simulink model "peacockElettricaSimulink2025b"  (R2025b)
settings: Solver=FixedStepAuto  StopTime=30  FixedStep=0.001  MaxStep=0.001
InitFcn:
  | run('setupParams.m');
StopFcn:
  | plot(out.X, out.Y); axis equal; grid on;
model workspace: external: MATLAB File (data not in the file)
values from neighbouring files (symbols this model uses):
  air_temp = 300    [setupParams.m]    (also in setupParamsSingle.m)
  brake_bias_f = 0.60    (= 0.6)    [setupParams.m]    (also in setupParamsSingle.m)
  brake_bias_r = 1 - brake_bias_f    (= 0.4)    [setupParams.m]    (also in setupParamsSingle.m)
  camber_front = -1.5    [setupParams.m]    (also in setupParamsSingle.m)
  camber_rear = -1    [setupParams.m]    (also in setupParamsSingle.m)
  g = 9.81    [setupParams.m]    (also in setupParamsSingle.m)
  gnd_displ = 0.0    (= 0)    [setupParams.m]    (also in setupParamsSingle.m)
  Kus = 0.00    (= 0)    [setupParams.m]    (also in setupParamsSingle.m)
  l_f = 0.775    [setupParams.m]    (also in setupParamsSingle.m)
  l_r = 0.775    [setupParams.m]    (also in setupParamsSingle.m)
  launch_ramp_rate = 1000.0    (= 1000)    [setupParams.m]    (also in setupParamsSingle.m)
  launch_V_thresh = 5.0    (= 5)    [setupParams.m]    (also in setupParamsSingle.m)
  mass = 300    [setupParams.m]    (also in setupParamsSingle.m)
  mu = 1.5    [setupParams.m]    (also in setupParamsSingle.m)
  nominal_ramp_rate = 1000.0    (= 1000)    [setupParams.m]    (also in setupParamsSingle.m)
  pa_front_wheel = 82700    [setupParams.m]    (also in setupParamsSingle.m)
  pa_rear_wheel = 82700    [setupParams.m]    (also in setupParamsSingle.m)
  pedal_bp = (0:10:100)'    [setupParams.m]    (also in setupParamsSingle.m)
  pedal_map = (pedal_bp / 100) .^ pedal_alpha    [setupParams.m]    (also in setupParamsSingle.m = (pedal_bp / 100) .^ pedal_alpha.Value)
  R_wheel = 0.2032    [setupParams.m]    (also in setupParamsSingle.m)
  regen_I_cont_A = 14.0    (= 14)    [setupParams.m]    (also in setupParamsSingle.m)
  regen_I_peak_A = 21.0    (= 21)    [setupParams.m]    (also in setupParamsSingle.m)
  regen_I_peak_dur_s = 4.0    (= 4)    [setupParams.m]    (also in setupParamsSingle.m)
  regen_P_batt_max_W = 35000    [setupParams.m]    (also in setupParamsSingle.m)
  regen_pedal_thr = 10.0    (= 10)    [setupParams.m]    (also in setupParamsSingle.m)
  regen_speed_crit_rpm = 2000    [setupParams.m]    (also in setupParamsSingle.m = 500)
  regen_speed_min_rpm = 4000    [setupParams.m]    (also in setupParamsSingle.m = 3000)
  regen_T_max = 5    [setupParams.m]    (also in setupParamsSingle.m = Simulink.Parameter(T_rated.Value/2))
  rid_eff = 0.80    (= 0.8)    [setupParams.m]    (also in setupParamsSingle.m)
  rid_ratio = 15    [setupParams.m]    (also in setupParamsSingle.m)
  scale_factor_front = ones(27, 1)    [setupParams.m]    (also in setupParamsSingle.m)
  scale_factor_rear = ones(27, 1)    [setupParams.m]    (also in setupParamsSingle.m)
  slc_Ki = 0    [setupParams.m]    (also in setupParamsSingle.m = Simulink.Parameter(0))
  slc_Kp = 0    [setupParams.m]    (also in setupParamsSingle.m = Simulink.Parameter(0))
  slc_low_sat = -T_peak    (= -21)    [setupParams.m]    (also in setupParamsSingle.m)
  slc_up_sat = T_peak    (= 21)    [setupParams.m]    (also in setupParamsSingle.m)
  slip_bc_coeff = 10    [setupParams.m]    (also in setupParamsSingle.m = Simulink.Parameter(1.5))
  slip_filt_N = 80    [setupParams.m]    (also in setupParamsSingle.m = 15)
  slip_Kd = 0.8    [setupParams.m]    (also in setupParamsSingle.m = Simulink.Parameter(5.0))
  slip_Ki = 13.0    (= 13)    [setupParams.m]    (also in setupParamsSingle.m = Simulink.Parameter(110.0))
  slip_Kp = 50.0    (= 50)    [setupParams.m]    (also in setupParamsSingle.m = Simulink.Parameter(180.0))
  slip_low_sat = 0.0    (= 0)    [setupParams.m]    (also in setupParamsSingle.m)
  slip_ref = 0.15    [setupParams.m]    (also in setupParamsSingle.m = Simulink.Parameter(0.15))
  slip_up_sat = 18    [setupParams.m]    (also in setupParamsSingle.m = 21)
  slip_V_min = 3    [setupParams.m]    (also in setupParamsSingle.m = 1)
  steer_ratio = 4.2    [pure_pursuit.m]    (also in setupParams.m; setupParamsSingle.m)
  T_headroom_max = 3.0    (= 3)    [setupParams.m]    (also in setupParamsSingle.m = Simulink.Parameter(5.0))
  T_peak = 21    [setupParams.m]    (also in setupParamsSingle.m)
  T_rated = 9.8    [setupParams.m]    (also in setupParamsSingle.m = Simulink.Parameter(9.8))
  track_width = (track_width_r + track_width_f)/2    (= 1.2)    [setupParams.m]    (also in setupParamsSingle.m = sqrt(track_width_r^2 + track_width_f^2))
  track_width_f = 1.2    [setupParams.m]    (also in setupParamsSingle.m)
  track_width_r = 1.2    [setupParams.m]    (also in setupParamsSingle.m)
  Ts = 0.01    [setupParams.m]    (also in setupParamsSingle.m)
  tvc_D_thresh = 0.060    (= 0.06)    [setupParams.m]    (also in setupParamsSingle.m)
  tvc_D_thresh_off = 0.03    [setupParams.m]    (also in setupParamsSingle.m)
  tvc_Kd = 8    [setupParams.m]    (also in setupParamsSingle.m = Simulink.Parameter(5))
  tvc_Ki = 250    [setupParams.m]    (also in setupParamsSingle.m = Simulink.Parameter(10))
  tvc_Kp = 650    [setupParams.m]    (also in setupParamsSingle.m = Simulink.Parameter(70))
  tvc_low_sat = Simulink.Parameter(0)    [setupParamsSingle.m]
  tvc_throttle_on = 3.0    (= 3)    [setupParams.m]    (also in setupParamsSingle.m = Simulink.Parameter(3.0))
  tvc_up_sat = Simulink.Parameter(T_peak)    [setupParamsSingle.m]
  tvc_V_off = 2.0    (= 2)    [setupParams.m]    (also in setupParamsSingle.m = Simulink.Parameter(2.0))
  tvc_V_on = 4.0    (= 4)    [setupParams.m]    (also in setupParamsSingle.m = Simulink.Parameter(4.0))
  tvc_yaw_thresh = 0.08    [setupParams.m]    (also in setupParamsSingle.m)
  tvc_yaw_thresh_off = 0.04    [setupParams.m]    (also in setupParamsSingle.m)
  v0_speed = 0.00    (= 0)    [setupParams.m]    (also in setupParamsSingle.m)
  V_dc = 540    [setupParams.m]    (also in setupParamsSingle.m)
  w_engine = 0.005    [setupParams.m]    (also in setupParamsSingle.m)
  wheelbase = l_f + l_r    (= 1.55)    [setupParams.m]    (also in setupParamsSingle.m)
libraries: simulink x12, slpidlib x4, vehdynlibtire x4, vehdynlibsteering x1, sim3dlib x1, sim3dautolib x1, autolibshared x1
(part 3 of 3)

== matlab function peacockElettricaSimulink2025b/DriveController/TVC/TorqueAllocator ==
  data: T_req input; T_RL_cmd output; dT input; derating_L input; derating_R input; T_RR_cmd output; D input; T_peak parameter; T_rated parameter; T_headroom_max parameter
% function [T_RL_cmd, T_RR_cmd] = fcn(T_req, dT, T_max_L, T_max_R, D)
%     T_min = 0;
%     T_headroom = min(5.0, 8.0 * abs(D));  % proporzionale allo sterzo
% 
%     T_lim_eff = min(T_max_L, T_max_R) - T_headroom;
%     T_req_eff = max(T_min, min(T_req, T_lim_eff));
% 
%     % Coppie desiderate
%     T_L = T_req_eff + dT;
%     T_R = T_req_eff - dT;
% 
%     % Saturazione superiore con yaw priority
%     if T_L > T_max_L
%         excess = T_L - T_max_L;
%         T_L = T_max_L;
%         T_R = T_R - excess;
%     end
%     if T_R > T_max_R
%         excess = T_R - T_max_R;
%         T_R = T_max_R;
%         T_L = T_L - excess;
%     end
% 
%     % Saturazione inferiore con yaw priority
%     if T_R < T_min
%         excess = T_min - T_R;
%         T_R = T_min;
%         T_L = T_L + excess;
%     end
%     if T_L < T_min
%         excess = T_min - T_L;
%         T_L = T_min;
%         T_R = T_R + excess;
%     end
% 
%     % Hard clip finale
%     T_L = max(T_min, min(T_max_L, T_L));
%     T_R = max(T_min, min(T_max_R, T_R));
% 
%     T_RL_cmd = T_L;
%     T_RR_cmd = T_R;
% end



function [T_RL_cmd, T_RR_cmd] = fcn(T_req, dT, derating_L, derating_R, D,T_peak, T_rated,T_headroom_max)
T_min    = 0;

% Stima T_max da bit di derating AMK status word
T_max_L = derating_L * T_rated + (1.0 - derating_L) * T_peak;
T_max_R = derating_R * T_rated + (1.0 - derating_R) * T_peak;

T_headroom = min(T_headroom_max, 8.0 * abs(D));
T_lim_eff = min(T_max_L, T_max_R) - T_headroom;
T_req_eff = max(T_min, min(T_req, T_lim_eff));

T_L = T_req_eff + dT;   % T_RL
T_R = T_req_eff - dT;   % T_RR

% Saturazione SENZA redistribuzione
T_L = max(T_min, min(T_max_L, T_L));
T_R = max(T_min, min(T_max_R, T_R));

T_RL_cmd = T_L;
T_RR_cmd = T_R;

end
